simulink model "static_fun_demo"  (R2014b)
settings: Solver=ode3  StartTime=0.0  StopTime=10.0  FixedStep=1e-3  RelTol=1e-3
libraries: periblklib x1
settings Model: Creator=Hyowinner  LastModifiedBy=Hyowinner
settings OptimizationCC: InlineParams=on  OptimizeModelRefInitCode=on  LifeSpan=1
settings RTWCC: SystemTargetFile=ert.tlc  GenCodeOnly=on  TemplateMakefile=ert_default_tmf  Description=Embedded Coder  GenerateReport=on  ProcessScript=ert_make_rtw_hook  IncludeHyperlinkInReport=on  LaunchReport=on
settings CodeAppCC: IgnoreCustomStorageClasses=off
settings ERTTargetCC: GenerateSampleERTMain=on  InlinedParameterPlacement=NonHierarchical  ERTCustomFileTemplate=example_file_process.tlc

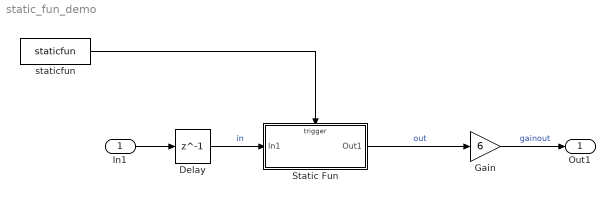
== system static_fun_demo ==
  In1 : Inport
  Delay : Delay  DelayLength=1  InitialCondition=0  StateName=in_old
      settings: CodeGenStateStorageClass=ExportedGlobal
  Gain : Gain  Gain=6
  Static Fun : Subsystem  TreatAsAtomicUnit=on
  staticfun : periblklib/Static Function/staticfun  g_fcnname=doTestStaticFunc
  Out1 : Outport
  wires:
  staticfun/1 -> Static Fun/Trigger
  In1/1 -> Delay/1
  Static Fun/1(Out1) -> Gain/1  "out"
  Gain/1 -> Out1/1  "gainout"
  Delay/1 -> Static Fun/1(In1)  "in"

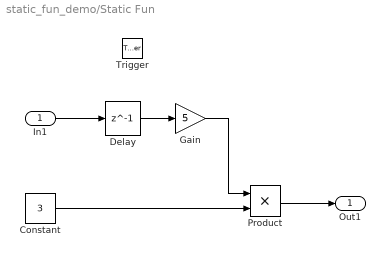
== system static_fun_demo/Static Fun ==
  In1 : Inport
  Trigger : TriggerPort  TriggerType=function-call  PortDimensions=1
  Constant : Constant  Value=3
  Delay : Delay  DelayLength=1  InitialCondition=0  StateName=old
      settings: CodeGenStateStorageClass=ExportedGlobal
  Gain : Gain  Gain=5
  Product : Product
  Out1 : Outport
  wires:
  Constant/1 -> Product/2
  In1/1 -> Delay/1
  Delay/1 -> Gain/1
  Gain/1 -> Product/1
  Product/1 -> Out1/1
